simulink model "The_Entire_Control_Algorithm"  (R2024b)
settings: Solver=FixedStepDiscrete  StartTime=0.0  StopTime=10.0  FixedStep=0.001  RelTol=1e-3
undefined symbols (not defined in the file or in its folder): dspblkCoreblockFVToolHelper, gcbh
libraries: arduinolib x21, slpidlib x6, simulink x5, sharedTrackingLibrary x1
(part 1 of 2)
settings Model: Creator=BU  LastModifiedBy=BU
settings OptimizationCC: DefaultParameterBehavior=Inlined  UseDivisionForNetSlopeComputation=on  GainParamInheritBuiltInType=on  UseFloatMulNetSlope=on  InlineInvariantSignals=on  PassReuseOutputArgsAs=Individual arguments  ZeroExternalMemoryAtStartup=off  ZeroInternalMemoryAtStartup=off  NoFixptDivByZeroProtection=on  EfficientFloat2IntCast=on  LifeSpan=1  OptimizeBlockOrder=speed  DifferentSizesBufferReuse=on  EfficientTunableParamExpr=on
settings DebuggingCC: ParameterTunabilityLossMsg=error
settings HardwareCC: ProdBitPerInt=16  ProdBitPerPointer=16  ProdBitPerSizeT=16  ProdBitPerPtrDiffT=16  ProdLargestAtomicFloat=None  ProdWordSize=16  ProdLongLongMode=on  ProdHWDeviceType=Atmel->AVR (8-bit)
settings SFSimCC: MATLABDynamicMemAlloc=off
settings RTWCC: Description=Embedded Coder  SystemTargetFile=ert.tlc  GenCodeOnly=on  TemplateMakefile=ert_default_tmf
settings CodeAppCC: ForceParamTrailComments=on  IgnoreCustomStorageClasses=off  OperatorAnnotations=on  SimulinkDataObjDesc=on  SFDataObjDesc=on  CustomSymbolStrGlobalVar=rt$N$M  CustomSymbolStrType=$N$M  CustomSymbolStrFcn=$N$M$F  CustomSymbolStrMacro=$N$M  InsertBlockDesc=on
settings ERTTargetCC: TargetLangStandard=C99 (ISO)  GenerateSampleERTMain=on  IncludeMdlTerminateFcn=off  CombineSignalStateStructs=on  SupportComplex=off  SupportContinuousTime=on  SupportNonInlinedSFcns=on  RootIOFormat=Structure reference  ERTCustomFileTemplate=example_file_process.tlc  ERTFilePackagingFormat=CompactWithDataFile

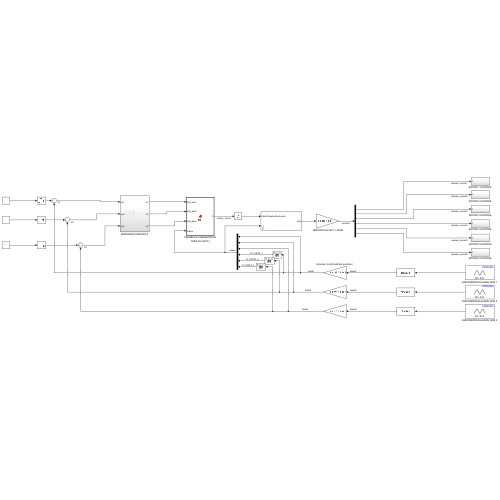
[thumbnail: Simulink's stored preview of the top-level diagram]
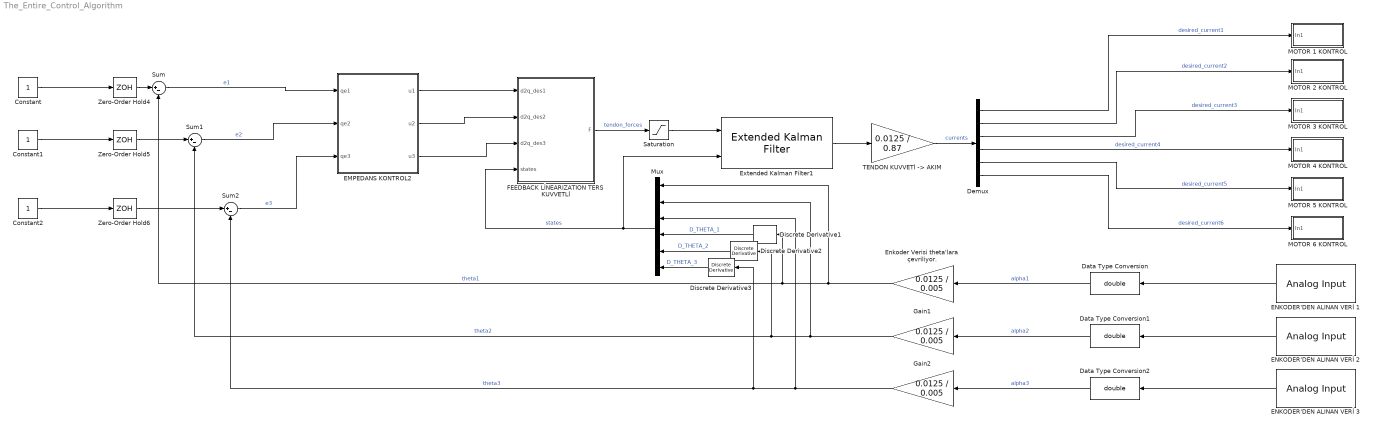
== system The_Entire_Control_Algorithm ==
  Constant : Constant
  Constant1 : Constant
  Constant2 : Constant
  Data Type Conversion : DataTypeConversion  OutDataTypeStr=double  SaturateOnIntegerOverflow=off  RndMeth=Floor
  Data Type Conversion1 : DataTypeConversion  OutDataTypeStr=double  SaturateOnIntegerOverflow=off  RndMeth=Floor
  Data Type Conversion2 : DataTypeConversion  OutDataTypeStr=double  SaturateOnIntegerOverflow=off  RndMeth=Floor
  Demux : Demux  Outputs=6
  Discrete Derivative1 : simulink/Discrete/Discrete Derivative  gainval=1.0  ICPrevScaledInput=0.0  OutMin=[]  OutMax=[]  OutDataType=fixdt(1, 16)  OutScaling=2^-10  DoSatur=off
  Discrete Derivative2 : simulink/Discrete/Discrete Derivative  gainval=1.0  ICPrevScaledInput=0.0  OutMin=[]  OutMax=[]  OutDataType=fixdt(1, 16)  OutScaling=2^-10  DoSatur=off
  Discrete Derivative3 : simulink/Discrete/Discrete Derivative  gainval=1.0  ICPrevScaledInput=0.0  OutMin=[]  OutMax=[]  OutDataType=fixdt(1, 16)  OutScaling=2^-10  DoSatur=off
  EMPEDANS KONTROL2 : Subsystem
  ENKODER'DEN ALINAN VERİ 1 : arduinolib/Analog Input  pinNumber=15  ReadResultsOnly=off  ConversionTriggerSource=Software  ExternalTriggerType=uint32( 0 )  OutputDataType=uint16  EnableConversionCompleteNotify=off  EnableOuputStatus=off  SampleTime=0.001  blockPlatform=arduino
  ENKODER'DEN ALINAN VERİ 2 : arduinolib/Analog Input  pinNumber=14  ReadResultsOnly=off  ConversionTriggerSource=Software  ExternalTriggerType=uint32( 0 )  OutputDataType=uint16  EnableConversionCompleteNotify=off  EnableOuputStatus=off  SampleTime=0.001  blockPlatform=arduino
  ENKODER'DEN ALINAN VERİ 3 : arduinolib/Analog Input  pinNumber=13  ReadResultsOnly=off  ConversionTriggerSource=Software  ExternalTriggerType=uint32( 0 )  OutputDataType=uint16  EnableConversionCompleteNotify=off  EnableOuputStatus=off  SampleTime=0.001  blockPlatform=arduino
  Enkoder Verisi theta'lara çevriliyor. : Gain  Gain=0.0125 / 0.005
  Extended Kalman Filter1 : sharedTrackingLibrary/Extended Kalman Filter  StateTransitionFcn=myStateTransitionFcn  HasStateTransitionJacobianFcn=off  StateTransitionJacobianFcn=0  HasAdditiveProcessNoise=Additive  ProcessNoise=diag([1e-7, 1e-7, 1e-7, 1e-7, 1e-7, 1e-7]);  HasTimeVaryingProcessNoise=off  HasStateTransitionFcnExtraArgument=1  InitialState=[0; 0; 0; 0; 0; 0]  InitialStateCovariance=[1e-6; 1e-6; 1e-6; 1e-6; 1e-6; 1e-6];  MeasurementFcn1=myMeasurementFcn  HasMeasurementJacobianFcn1=off  HasMeasurementEnablePort1=off  HasAdditiveMeasurementNoise1=Additive  MeasurementNoise1=[1e-1; 1e-1; 1e-1; 1e-1; 1e-1; 1e-1];  HasTimeVaryingMeasurementNoise1=off  HasMeasurementFcnExtraArgument1=0  HasMeasurementWrapping1=off  MeasurementFcn2=myMeasurementFcn  HasMeasurementJacobianFcn2=off  HasMeasurementEnablePort2=off  HasAdditiveMeasurementNoise2=Additive  MeasurementNoise2=1  HasTimeVaryingMeasurementNoise2=off  HasMeasurementFcnExtraArgument2=0  HasMeasurementWrapping2=off  MeasurementFcn3=myMeasurementFcn  HasMeasurementJacobianFcn3=off  HasMeasurementEnablePort3=off  HasAdditiveMeasurementNoise3=Additive  MeasurementNoise3=1  HasTimeVaryingMeasurementNoise3=off  HasMeasurementFcnExtraArgument3=0  HasMeasurementWrapping3=off  MeasurementFcn4=myMeasurementFcn  HasMeasurementJacobianFcn4=off  HasMeasurementEnablePort4=off  HasAdditiveMeasurementNoise4=Additive  MeasurementNoise4=1  HasTimeVaryingMeasurementNoise4=off  HasMeasurementFcnExtraArgument4=0  HasMeasurementWrapping4=off  MeasurementFcn5=myMeasurementFcn  HasMeasurementJacobianFcn5=off  HasMeasurementEnablePort5=off  HasAdditiveMeasurementNoise5=Additive  MeasurementNoise5=1  HasTimeVaryingMeasurementNoise5=off  HasMeasurementFcnExtraArgument5=0  HasMeasurementWrapping5=off  EnableMultirate=off  StateTransitionFcnSampleTime=1  MeasurementFcn1SampleTime=1  MeasurementFcn2SampleTime=1  MeasurementFcn3SampleTime=1  MeasurementFcn4SampleTime=1  MeasurementFcn5SampleTime=1  UseCurrentEstimator=on  OutputStateCovariance=off  DataType=double  SampleTime=0.001  NumberOfMeasurements=1
      settings: LibrarySourceBlock=slident/Estimators/Extended Kalman Filter
  FEEDBACK LİNEARIZATION TERS KUVVETLİ : MATLAB Function  TreatAsAtomicUnit=on
  Gain1 : Gain  Gain=0.0125 / 0.005
  Gain2 : Gain  Gain=0.0125 / 0.005
  MOTOR 1 KONTROL : Subsystem
  MOTOR 2 KONTROL : Subsystem
  MOTOR 3 KONTROL : Subsystem
  MOTOR 4 KONTROL : Subsystem
  MOTOR 5 KONTROL : Subsystem
  MOTOR 6 KONTROL : Subsystem
  Mux : Mux  Inputs=6
  Saturation : Saturate  UpperLimit=7  LowerLimit=-7
  Sum : Sum  Inputs=|+-
  Sum1 : Sum  Inputs=|+-
  Sum2 : Sum  Inputs=|+-
  "TENDON KUVVETİ -> AKIM" : Gain  Gain=0.0125 / 0.87
  Zero-Order Hold4 : ZeroOrderHold  SampleTime=0.001
  Zero-Order Hold5 : ZeroOrderHold  SampleTime=0.001
  Zero-Order Hold6 : ZeroOrderHold  SampleTime=0.001
  wires:
  Demux/5 -> MOTOR 5 KONTROL/1(In1)  "desired_current5"
  Demux/4 -> MOTOR 4 KONTROL/1(In1)  "desired_current4"
  Demux/6 -> MOTOR 6 KONTROL/1(In1)  "desired_current6"
  Demux/2 -> MOTOR 2 KONTROL/1(In1)  "desired_current2"
  Demux/3 -> MOTOR 3 KONTROL/1(In1)  "desired_current3"
  ENKODER'DEN ALINAN VERİ 3/1 -> Data Type Conversion2/1
  ENKODER'DEN ALINAN VERİ 1/1 -> Data Type Conversion/1
  ENKODER'DEN ALINAN VERİ 2/1 -> Data Type Conversion1/1
  Demux/1 -> MOTOR 1 KONTROL/1(In1)  "desired_current1"
  Discrete Derivative1/1 -> Mux/4  "D_THETA_1"
  Discrete Derivative2/1 -> Mux/5  "D_THETA_2"
  Discrete Derivative3/1 -> Mux/6  "D_THETA_3"
  Data Type Conversion/1 -> Enkoder Verisi theta'lara çevriliyor./1  "alpha1"
  Data Type Conversion1/1 -> Gain1/1  "alpha2"
  Data Type Conversion2/1 -> Gain2/1  "alpha3"
  "TENDON KUVVETİ -> AKIM"/1 -> Demux/1  "currents"
  Enkoder Verisi theta'lara çevriliyor./1 -> Sum/2, Discrete Derivative1/1, Mux/1  "theta1"
  Gain1/1 -> Sum1/2, Discrete Derivative2/1, Mux/2  "theta2"
  Gain2/1 -> Sum2/2, Discrete Derivative3/1, Mux/3  "theta3"
  Zero-Order Hold4/1 -> Sum/1
  EMPEDANS KONTROL2/2(u2) -> FEEDBACK LİNEARIZATION TERS KUVVETLİ/2(d2q_des2)
  Sum/1 -> EMPEDANS KONTROL2/1(qe1)  "e1"
  Sum1/1 -> EMPEDANS KONTROL2/2(qe2)  "e2"
  Sum2/1 -> EMPEDANS KONTROL2/3(qe3)  "e3"
  Zero-Order Hold6/1 -> Sum2/1
  Constant1/1 -> Zero-Order Hold5/1
  FEEDBACK LİNEARIZATION TERS KUVVETLİ/1(F) -> Saturation/1  "tendon_forces"
  Zero-Order Hold5/1 -> Sum1/1
  EMPEDANS KONTROL2/1(u1) -> FEEDBACK LİNEARIZATION TERS KUVVETLİ/1(d2q_des1)
  Constant2/1 -> Zero-Order Hold6/1
  EMPEDANS KONTROL2/3(u3) -> FEEDBACK LİNEARIZATION TERS KUVVETLİ/3(d2q_des3)
  Constant/1 -> Zero-Order Hold4/1
  Mux/1 -> Extended Kalman Filter1/2, FEEDBACK LİNEARIZATION TERS KUVVETLİ/4(states)  "states"
  Saturation/1 -> Extended Kalman Filter1/1
  Extended Kalman Filter1/1 -> "TENDON KUVVETİ -> AKIM"/1

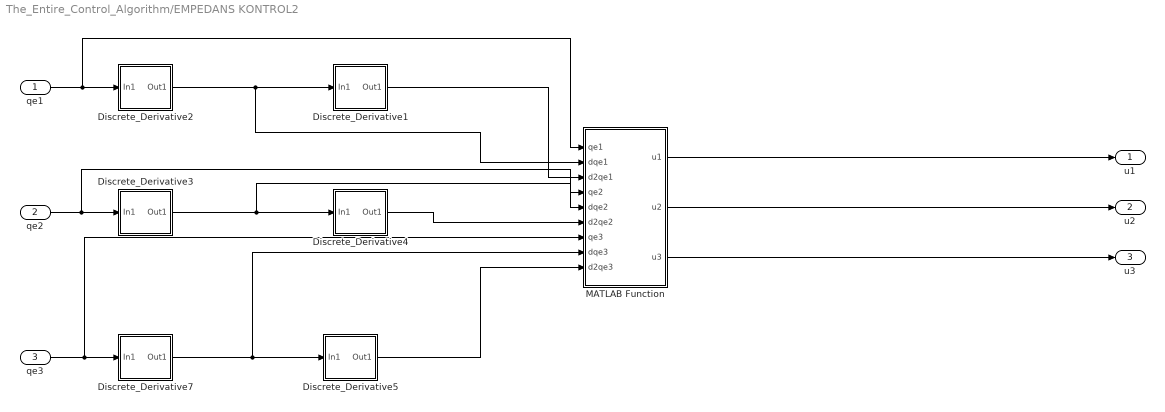
== system The_Entire_Control_Algorithm/EMPEDANS KONTROL2 ==
  qe1 : Inport
  qe2 : Inport  Port=2
  qe3 : Inport  Port=3
  Discrete_Derivative1 : Subsystem
  Discrete_Derivative2 : Subsystem
  Discrete_Derivative3 : Subsystem
  Discrete_Derivative4 : Subsystem
  Discrete_Derivative5 : Subsystem
  Discrete_Derivative7 : Subsystem
  MATLAB Function : MATLAB Function  TreatAsAtomicUnit=on
  u1 : Outport
  u2 : Outport  Port=2
  u3 : Outport  Port=3
  wires:
  qe1/1 -> Discrete_Derivative2/1(In1), MATLAB Function/1(qe1)
  qe2/1 -> Discrete_Derivative3/1(In1), MATLAB Function/4(qe2)
  qe3/1 -> Discrete_Derivative7/1(In1), MATLAB Function/7(qe3)
  Discrete_Derivative2/1(Out1) -> Discrete_Derivative1/1(In1), MATLAB Function/2(dqe1)
  Discrete_Derivative3/1(Out1) -> Discrete_Derivative4/1(In1), MATLAB Function/5(dqe2)
  Discrete_Derivative7/1(Out1) -> Discrete_Derivative5/1(In1), MATLAB Function/8(dqe3)
  Discrete_Derivative1/1(Out1) -> MATLAB Function/3(d2qe1)
  Discrete_Derivative4/1(Out1) -> MATLAB Function/6(d2qe2)
  Discrete_Derivative5/1(Out1) -> MATLAB Function/9(d2qe3)
  MATLAB Function/1(u1) -> u1/1
  MATLAB Function/2(u2) -> u2/1
  MATLAB Function/3(u3) -> u3/1

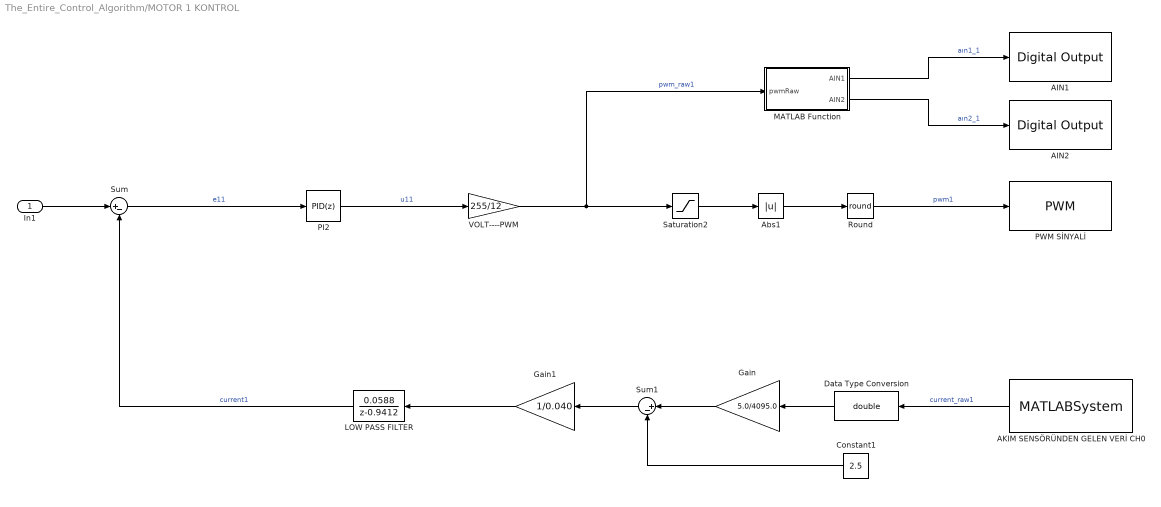
== system The_Entire_Control_Algorithm/MOTOR 1 KONTROL ==
  In1 : Inport
  AIN1 : arduinolib/Digital Output  pinNumber=24  Direction=output  blockPlatform=arduino
  AIN2 : arduinolib/Digital Output  pinNumber=25  Direction=output  blockPlatform=arduino
  AKIM SENSÖRÜNDEN GELEN VERİ CH0 : MATLABSystem  System=MCP3208Reader  Channel=0  SimulateUsing=Code generation
      mask Type: MCP3208Reader
      mask Display:
      | disp('MCP3208Reader');
      | port_label('output',1,'value');
  Abs1 : Abs  RndMeth=Round  SaturateOnIntegerOverflow=off
  Constant1 : Constant  Value=2.5
  Data Type Conversion : DataTypeConversion  OutDataTypeStr=double  SaturateOnIntegerOverflow=off  RndMeth=Floor
  Gain : Gain  Gain=5.0/4095.0
  Gain1 : Gain  Gain=1/0.040
  LOW PASS FILTER : DiscreteTransferFcn  LoadFcn=dspblkCoreblockFVToolHelper(gcbh,'load');  Numerator=[0.0588]  Denominator=[1 -0.9412]
      settings: CopyFcn=dspblkCoreblockFVToolHelper(gcbh,'copy');  DeleteFcn=dspblkCoreblockFVToolHelper(gcbh,'close');  ModelCloseFcn=dspblkCoreblockFVToolHelper(gcbh,'close');  PreSaveFcn=dspblkCoreblockFVToolHelper(gcbh,'presave');  PostSaveFcn=dspblkCoreblockFVToolHelper(gcbh,'postsave');  CloseFcn=dspblkCoreblockFVToolHelper(gcbh,'close');
  MATLAB Function : MATLAB Function  TreatAsAtomicUnit=on
  PI2 : slpidlib/PID Controller  Controller=PID  Form=Parallel  TimeDomain=Discrete-time  UseExternalTs=off  SampleTime=0.001  IntegratorMethod=Forward Euler  FilterMethod=Forward Euler  ControllerParametersSource=internal  P=21  I=900  UseKiTs=off  D=0  UseExternalDerivativeSource=off  N=100  UseFilter=off  TunerSelectOption=Transfer Function Based (PID Tuner App)  InitialConditionSource=internal  InitialConditionForIntegrator=0  InitialConditionForFilter=0  DifferentiatorICPrevScaledInput=0  ExternalReset=none  TrackingMode=off  Kt=1  LimitOutput=off  SatLimitsSource=internal  UpperSaturationLimit=inf  LowerSaturationLimit=-inf  LinearizeAsGain=on  AntiWindupMode=none  Kb=1  LimitIntegrator=off  UpperIntegratorSaturationLimit=inf  LowerIntegratorSaturationLimit=-inf  POutMin=[]  POutMax=[]  IOutMin=[]  IOutMax=[]  DOutMin=[]  DOutMax=[]  NOutMin=[]  NOutMax=[]  SumOutMin=[]  SumOutMax=[]  SaturationOutMin=[]  SaturationOutMax=[]  PParamMin=[]  PParamMax=[]  IParamMin=[]  IParamMax=[]  DParamMin=[]  DParamMax=[]  NParamMin=[]  NParamMax=[]  KbParamMin=[]  KbParamMax=[]  KtParamMin=[]  KtParamMax=[]  KbOutMin=[]  KbOutMax=[]  KtOutMin=[]  KtOutMax=[]  IntegratorOutMin=[]  IntegratorOutMax=[]  FilterOutMin=[]  FilterOutMax=[]  SumI1OutMin=[]  SumI1OutMax=[]  SumI2OutMin=[]  SumI2OutMax=[]  SumI3OutMin=[]  SumI3OutMax=[]  SumI4OutMin=[]  SumI4OutMax=[]  SumDOutMin=[]  SumDOutMax=[]  DifferentiatorOutMin=[]  DifferentiatorOutMax=[]  FilterDiffOutCoefMin=[]  FilterDiffOutCoefMax=[]  ReciprocalOutMin=[]  ReciprocalOutMax=[]  SumDenOutMin=[]  SumDenOutMax=[]  SumNumOutMin=[]  SumNumOutMax=[]  DivideOutMin=[]  DivideOutMax=[]  UdiffTsProdOutMin=[]  UdiffTsProdOutMax=[]  NTsProdOutMin=[]  NTsProdOutMax=[]  UintegralTsProdOutMin=[]  UintegralTsProdOutMax=[]  UngainTsProdOutMin=[]  UngainTsProdOutMax=[]  ClampingZeroOutDataTypeStr=Inherit: Inherit via back propagation  ClampingZeroOutMin=[]  ClampingZeroOutMax=[]  FilterDenConstantOutDataTypeStr=Inherit: Inherit via back propagation  FilterDenConstantOutMin=[]  FilterDenConstantOutMax=[]  PCopyOutDataTypeStr=Inherit: Inherit via back propagation  PCopyOutMin=[]  PCopyOutMax=[]  NCopyOutDataTypeStr=Inherit: Inherit via back propagation  NCopyOutMin=[]  NCopyOutMax=[]  IntegratorContinuousStateAttributes=''  IntegratorStateMustResolveToSignalObject=off  IntegratorRTWStateStorageClass=Auto  FilterContinuousStateAttributes=''  FilterStateMustResolveToSignalObject=off  FilterRTWStateStorageClass=Auto  ParallelPVariant=InternalParameters  IdealPVariant=Disabled  IVariant=InternalParameters  DVariant=InternalParameters  IntegratorVariant=Discrete  SatVariant=Disabled  AWVariant=Passthrough  PCopyVariant=Disabled  TRVariant=Disabled  FdbkBlocksVariant=Forward  IdealPFdbkVariant=Disabled  SatFdbkVariant=Disabled  DerivativeFilterVariant=Differentiator  NVariant=Passthrough  NCopyVariant=Disabled_SignalSpec  FilterICVariant=InternalICsDifferentiator  IntegratorICVariant=InternalICs  ExternalResetVariant=Disabled  TRSumVariant=Passthrough  SumFdbkVariant=Disabled  SumVariant=Sum_PID  TsampFilterVariant=InternalTs  TsampNgainVariant=Passthrough  TsampIntegralVariant=Disabled_SignalSpec  ExternalSaturationOutDataTypeStr=Inherit: Same as second input  DerivativeSourceVariant=ErrorSignal  PreIntVariant=InternalPreInt
  PWM SİNYALİ : arduinolib/PWM  pinNumber=2  frequencyType=Default  desiredFrequency=490  achievableFrequency=490.2
  Round : Rounding  Operator=round
  Saturation2 : Saturate  UpperLimit=255  LowerLimit=-255
  Sum : Sum  Inputs=|+-
  Sum1 : Sum  Inputs=|+-
  VOLT----PWM : Gain  Gain=255/12
  wires:
  Gain1/1 -> LOW PASS FILTER/1
  VOLT----PWM/1 -> MATLAB Function/1(pwmRaw), Saturation2/1  "pwm_raw1"
  MATLAB Function/2(AIN2) -> AIN2/1  "aın2_1"
  Saturation2/1 -> Abs1/1
  Sum1/1 -> Gain1/1
  PI2/1 -> VOLT----PWM/1  "u11"
  In1/1 -> Sum/1
  LOW PASS FILTER/1 -> Sum/2  "current1"
  Round/1 -> PWM SİNYALİ/1  "pwm1"
  Constant1/1 -> Sum1/2
  AKIM SENSÖRÜNDEN GELEN VERİ CH0/1 -> Data Type Conversion/1  "current_raw1"
  Gain/1 -> Sum1/1
  Abs1/1 -> Round/1
  Sum/1 -> PI2/1  "e11"
  MATLAB Function/1(AIN1) -> AIN1/1  "aın1_1"
  Data Type Conversion/1 -> Gain/1

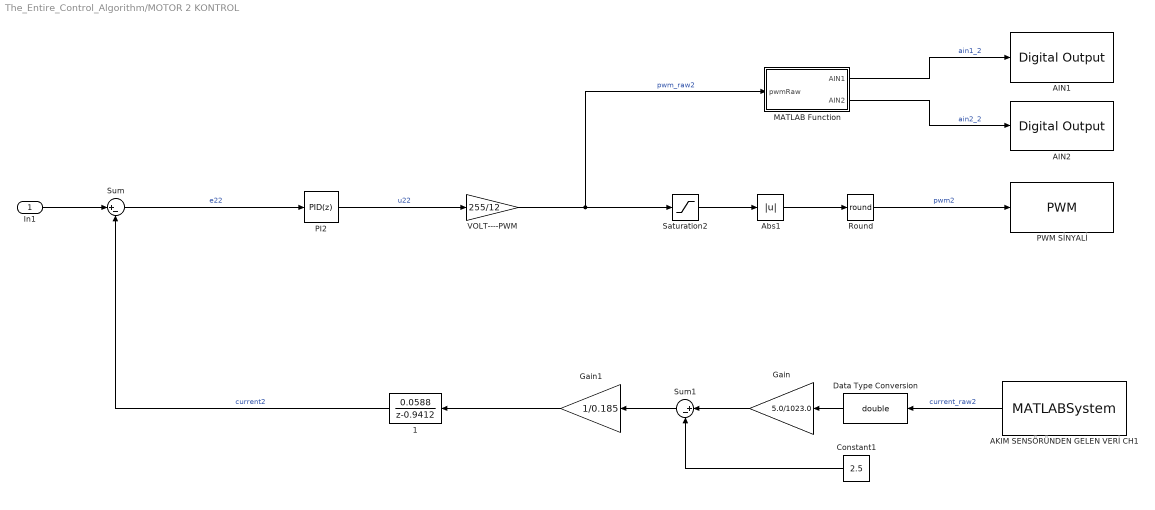
== system The_Entire_Control_Algorithm/MOTOR 2 KONTROL ==
  In1 : Inport
  1 : DiscreteTransferFcn  LoadFcn=dspblkCoreblockFVToolHelper(gcbh,'load');  Numerator=[0.0588]  Denominator=[1 -0.9412]
      settings: CopyFcn=dspblkCoreblockFVToolHelper(gcbh,'copy');  DeleteFcn=dspblkCoreblockFVToolHelper(gcbh,'close');  ModelCloseFcn=dspblkCoreblockFVToolHelper(gcbh,'close');  PreSaveFcn=dspblkCoreblockFVToolHelper(gcbh,'presave');  PostSaveFcn=dspblkCoreblockFVToolHelper(gcbh,'postsave');  CloseFcn=dspblkCoreblockFVToolHelper(gcbh,'close');
  AIN1 : arduinolib/Digital Output  pinNumber=26  Direction=output  blockPlatform=arduino
  AIN2 : arduinolib/Digital Output  pinNumber=27  Direction=output  blockPlatform=arduino
  AKIM SENSÖRÜNDEN GELEN VERİ CH1 : MATLABSystem  System=MCP3208Reader  Channel=0  SimulateUsing=Code generation
      mask Type: MCP3208Reader
      mask Display:
      | disp('MCP3208Reader');
      | port_label('output',1,'value');
  Abs1 : Abs  RndMeth=Round  SaturateOnIntegerOverflow=off
  Constant1 : Constant  Value=2.5
  Data Type Conversion : DataTypeConversion  OutDataTypeStr=double  SaturateOnIntegerOverflow=off  RndMeth=Floor
  Gain : Gain  Gain=5.0/1023.0
  Gain1 : Gain  Gain=1/0.185
  MATLAB Function : MATLAB Function  TreatAsAtomicUnit=on
  PI2 : slpidlib/PID Controller  Controller=PID  Form=Parallel  TimeDomain=Discrete-time  UseExternalTs=off  SampleTime=0.001  IntegratorMethod=Forward Euler  FilterMethod=Forward Euler  ControllerParametersSource=internal  P=21  I=900  UseKiTs=off  D=0.15  UseExternalDerivativeSource=off  N=100  UseFilter=off  TunerSelectOption=Transfer Function Based (PID Tuner App)  InitialConditionSource=internal  InitialConditionForIntegrator=0  InitialConditionForFilter=0  DifferentiatorICPrevScaledInput=0  ExternalReset=none  TrackingMode=off  Kt=1  LimitOutput=off  SatLimitsSource=internal  UpperSaturationLimit=inf  LowerSaturationLimit=-inf  LinearizeAsGain=on  AntiWindupMode=none  Kb=1  LimitIntegrator=off  UpperIntegratorSaturationLimit=inf  LowerIntegratorSaturationLimit=-inf  POutMin=[]  POutMax=[]  IOutMin=[]  IOutMax=[]  DOutMin=[]  DOutMax=[]  NOutMin=[]  NOutMax=[]  SumOutMin=[]  SumOutMax=[]  SaturationOutMin=[]  SaturationOutMax=[]  PParamMin=[]  PParamMax=[]  IParamMin=[]  IParamMax=[]  DParamMin=[]  DParamMax=[]  NParamMin=[]  NParamMax=[]  KbParamMin=[]  KbParamMax=[]  KtParamMin=[]  KtParamMax=[]  KbOutMin=[]  KbOutMax=[]  KtOutMin=[]  KtOutMax=[]  IntegratorOutMin=[]  IntegratorOutMax=[]  FilterOutMin=[]  FilterOutMax=[]  SumI1OutMin=[]  SumI1OutMax=[]  SumI2OutMin=[]  SumI2OutMax=[]  SumI3OutMin=[]  SumI3OutMax=[]  SumI4OutMin=[]  SumI4OutMax=[]  SumDOutMin=[]  SumDOutMax=[]  DifferentiatorOutMin=[]  DifferentiatorOutMax=[]  FilterDiffOutCoefMin=[]  FilterDiffOutCoefMax=[]  ReciprocalOutMin=[]  ReciprocalOutMax=[]  SumDenOutMin=[]  SumDenOutMax=[]  SumNumOutMin=[]  SumNumOutMax=[]  DivideOutMin=[]  DivideOutMax=[]  UdiffTsProdOutMin=[]  UdiffTsProdOutMax=[]  NTsProdOutMin=[]  NTsProdOutMax=[]  UintegralTsProdOutMin=[]  UintegralTsProdOutMax=[]  UngainTsProdOutMin=[]  UngainTsProdOutMax=[]  ClampingZeroOutDataTypeStr=Inherit: Inherit via back propagation  ClampingZeroOutMin=[]  ClampingZeroOutMax=[]  FilterDenConstantOutDataTypeStr=Inherit: Inherit via back propagation  FilterDenConstantOutMin=[]  FilterDenConstantOutMax=[]  PCopyOutDataTypeStr=Inherit: Inherit via back propagation  PCopyOutMin=[]  PCopyOutMax=[]  NCopyOutDataTypeStr=Inherit: Inherit via back propagation  NCopyOutMin=[]  NCopyOutMax=[]  IntegratorContinuousStateAttributes=''  IntegratorStateMustResolveToSignalObject=off  IntegratorRTWStateStorageClass=Auto  FilterContinuousStateAttributes=''  FilterStateMustResolveToSignalObject=off  FilterRTWStateStorageClass=Auto  ParallelPVariant=InternalParameters  IdealPVariant=Disabled  IVariant=InternalParameters  DVariant=InternalParameters  IntegratorVariant=Discrete  SatVariant=Disabled  AWVariant=Passthrough  PCopyVariant=Disabled  TRVariant=Disabled  FdbkBlocksVariant=Forward  IdealPFdbkVariant=Disabled  SatFdbkVariant=Disabled  DerivativeFilterVariant=Differentiator  NVariant=Passthrough  NCopyVariant=Disabled_SignalSpec  FilterICVariant=InternalICsDifferentiator  IntegratorICVariant=InternalICs  ExternalResetVariant=Disabled  TRSumVariant=Passthrough  SumFdbkVariant=Disabled  SumVariant=Sum_PID  TsampFilterVariant=InternalTs  TsampNgainVariant=Passthrough  TsampIntegralVariant=Disabled_SignalSpec  ExternalSaturationOutDataTypeStr=Inherit: Same as second input  DerivativeSourceVariant=ErrorSignal  PreIntVariant=InternalPreInt
  PWM SİNYALİ : arduinolib/PWM  pinNumber=3  frequencyType=Specify  desiredFrequency=490  achievableFrequency=490.2
  Round : Rounding  Operator=round
  Saturation2 : Saturate  UpperLimit=255  LowerLimit=-255
  Sum : Sum  Inputs=|+-
  Sum1 : Sum  Inputs=|+-
  VOLT----PWM : Gain  Gain=255/12
  wires:
  In1/1 -> Sum/1
  MATLAB Function/1(AIN1) -> AIN1/1  "ain1_2"
  Sum/1 -> PI2/1  "e22"
  Constant1/1 -> Sum1/2
  Round/1 -> PWM SİNYALİ/1  "pwm2"
  Gain/1 -> Sum1/1
  Abs1/1 -> Round/1
  1/1 -> Sum/2  "current2"
  VOLT----PWM/1 -> MATLAB Function/1(pwmRaw), Saturation2/1  "pwm_raw2"
  MATLAB Function/2(AIN2) -> AIN2/1  "ain2_2"
  Saturation2/1 -> Abs1/1
  Gain1/1 -> 1/1
  Sum1/1 -> Gain1/1
  PI2/1 -> VOLT----PWM/1  "u22"
  Data Type Conversion/1 -> Gain/1
  AKIM SENSÖRÜNDEN GELEN VERİ CH1/1 -> Data Type Conversion/1  "current_raw2"

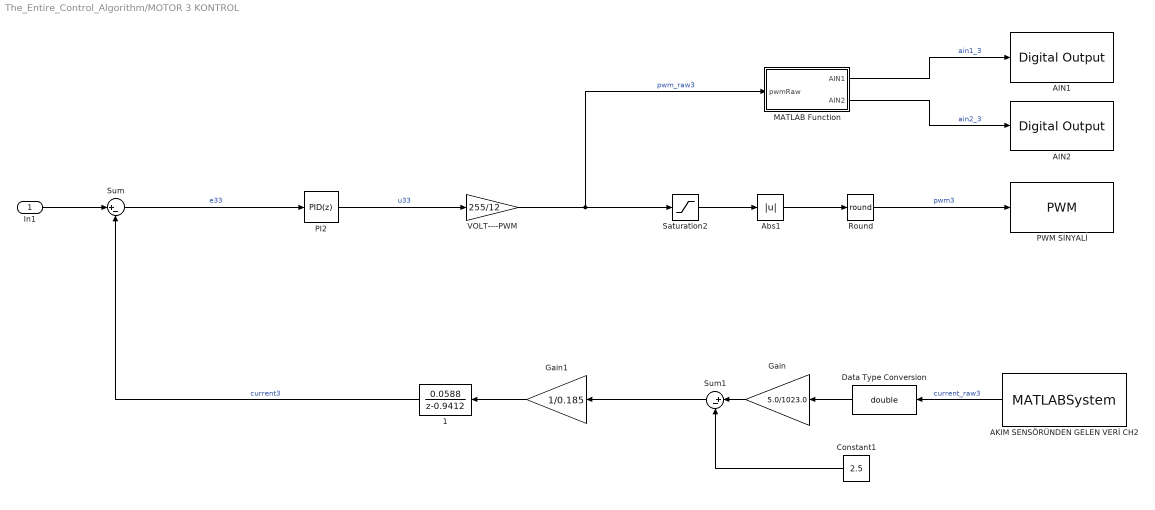
== system The_Entire_Control_Algorithm/MOTOR 3 KONTROL ==
  In1 : Inport
  1 : DiscreteTransferFcn  LoadFcn=dspblkCoreblockFVToolHelper(gcbh,'load');  Numerator=[0.0588]  Denominator=[1 -0.9412]
      settings: CopyFcn=dspblkCoreblockFVToolHelper(gcbh,'copy');  DeleteFcn=dspblkCoreblockFVToolHelper(gcbh,'close');  ModelCloseFcn=dspblkCoreblockFVToolHelper(gcbh,'close');  PreSaveFcn=dspblkCoreblockFVToolHelper(gcbh,'presave');  PostSaveFcn=dspblkCoreblockFVToolHelper(gcbh,'postsave');  CloseFcn=dspblkCoreblockFVToolHelper(gcbh,'close');
  AIN1 : arduinolib/Digital Output  pinNumber=28  Direction=output  blockPlatform=arduino
  AIN2 : arduinolib/Digital Output  pinNumber=29  Direction=output  blockPlatform=arduino
  AKIM SENSÖRÜNDEN GELEN VERİ CH2 : MATLABSystem  System=MCP3208Reader  Channel=0  SimulateUsing=Code generation
      mask Type: MCP3208Reader
      mask Display:
      | disp('MCP3208Reader');
      | port_label('output',1,'value');
  Abs1 : Abs  RndMeth=Round  SaturateOnIntegerOverflow=off
  Constant1 : Constant  Value=2.5
  Data Type Conversion : DataTypeConversion  OutDataTypeStr=double  SaturateOnIntegerOverflow=off  RndMeth=Floor
  Gain : Gain  Gain=5.0/1023.0
  Gain1 : Gain  Gain=1/0.185
  MATLAB Function : MATLAB Function  TreatAsAtomicUnit=on
  PI2 : slpidlib/PID Controller  Controller=PID  Form=Parallel  TimeDomain=Discrete-time  UseExternalTs=off  SampleTime=0.001  IntegratorMethod=Forward Euler  FilterMethod=Forward Euler  ControllerParametersSource=internal  P=21  I=900  UseKiTs=off  D=0.15  UseExternalDerivativeSource=off  N=100  UseFilter=off  TunerSelectOption=Transfer Function Based (PID Tuner App)  InitialConditionSource=internal  InitialConditionForIntegrator=0  InitialConditionForFilter=0  DifferentiatorICPrevScaledInput=0  ExternalReset=none  TrackingMode=off  Kt=1  LimitOutput=off  SatLimitsSource=internal  UpperSaturationLimit=inf  LowerSaturationLimit=-inf  LinearizeAsGain=on  AntiWindupMode=none  Kb=1  LimitIntegrator=off  UpperIntegratorSaturationLimit=inf  LowerIntegratorSaturationLimit=-inf  POutMin=[]  POutMax=[]  IOutMin=[]  IOutMax=[]  DOutMin=[]  DOutMax=[]  NOutMin=[]  NOutMax=[]  SumOutMin=[]  SumOutMax=[]  SaturationOutMin=[]  SaturationOutMax=[]  PParamMin=[]  PParamMax=[]  IParamMin=[]  IParamMax=[]  DParamMin=[]  DParamMax=[]  NParamMin=[]  NParamMax=[]  KbParamMin=[]  KbParamMax=[]  KtParamMin=[]  KtParamMax=[]  KbOutMin=[]  KbOutMax=[]  KtOutMin=[]  KtOutMax=[]  IntegratorOutMin=[]  IntegratorOutMax=[]  FilterOutMin=[]  FilterOutMax=[]  SumI1OutMin=[]  SumI1OutMax=[]  SumI2OutMin=[]  SumI2OutMax=[]  SumI3OutMin=[]  SumI3OutMax=[]  SumI4OutMin=[]  SumI4OutMax=[]  SumDOutMin=[]  SumDOutMax=[]  DifferentiatorOutMin=[]  DifferentiatorOutMax=[]  FilterDiffOutCoefMin=[]  FilterDiffOutCoefMax=[]  ReciprocalOutMin=[]  ReciprocalOutMax=[]  SumDenOutMin=[]  SumDenOutMax=[]  SumNumOutMin=[]  SumNumOutMax=[]  DivideOutMin=[]  DivideOutMax=[]  UdiffTsProdOutMin=[]  UdiffTsProdOutMax=[]  NTsProdOutMin=[]  NTsProdOutMax=[]  UintegralTsProdOutMin=[]  UintegralTsProdOutMax=[]  UngainTsProdOutMin=[]  UngainTsProdOutMax=[]  ClampingZeroOutDataTypeStr=Inherit: Inherit via back propagation  ClampingZeroOutMin=[]  ClampingZeroOutMax=[]  FilterDenConstantOutDataTypeStr=Inherit: Inherit via back propagation  FilterDenConstantOutMin=[]  FilterDenConstantOutMax=[]  PCopyOutDataTypeStr=Inherit: Inherit via back propagation  PCopyOutMin=[]  PCopyOutMax=[]  NCopyOutDataTypeStr=Inherit: Inherit via back propagation  NCopyOutMin=[]  NCopyOutMax=[]  IntegratorContinuousStateAttributes=''  IntegratorStateMustResolveToSignalObject=off  IntegratorRTWStateStorageClass=Auto  FilterContinuousStateAttributes=''  FilterStateMustResolveToSignalObject=off  FilterRTWStateStorageClass=Auto  ParallelPVariant=InternalParameters  IdealPVariant=Disabled  IVariant=InternalParameters  DVariant=InternalParameters  IntegratorVariant=Discrete  SatVariant=Disabled  AWVariant=Passthrough  PCopyVariant=Disabled  TRVariant=Disabled  FdbkBlocksVariant=Forward  IdealPFdbkVariant=Disabled  SatFdbkVariant=Disabled  DerivativeFilterVariant=Differentiator  NVariant=Passthrough  NCopyVariant=Disabled_SignalSpec  FilterICVariant=InternalICsDifferentiator  IntegratorICVariant=InternalICs  ExternalResetVariant=Disabled  TRSumVariant=Passthrough  SumFdbkVariant=Disabled  SumVariant=Sum_PID  TsampFilterVariant=InternalTs  TsampNgainVariant=Passthrough  TsampIntegralVariant=Disabled_SignalSpec  ExternalSaturationOutDataTypeStr=Inherit: Same as second input  DerivativeSourceVariant=ErrorSignal  PreIntVariant=InternalPreInt
  PWM SİNYALİ : arduinolib/PWM  pinNumber=4  frequencyType=Default  desiredFrequency=490  achievableFrequency=490.2
  Round : Rounding  Operator=round
  Saturation2 : Saturate  UpperLimit=255  LowerLimit=-255
  Sum : Sum  Inputs=|+-
  Sum1 : Sum  Inputs=|+-
  VOLT----PWM : Gain  Gain=255/12
  wires:
  In1/1 -> Sum/1
  Gain1/1 -> 1/1
  Saturation2/1 -> Abs1/1
  PI2/1 -> VOLT----PWM/1  "u33"
  MATLAB Function/2(AIN2) -> AIN2/1  "ain2_3"
  Sum1/1 -> Gain1/1
  Gain/1 -> Sum1/1
  VOLT----PWM/1 -> MATLAB Function/1(pwmRaw), Saturation2/1  "pwm_raw3"
  Abs1/1 -> Round/1
  1/1 -> Sum/2  "current3"
  Sum/1 -> PI2/1  "e33"
  Round/1 -> PWM SİNYALİ/1  "pwm3"
  Constant1/1 -> Sum1/2
  MATLAB Function/1(AIN1) -> AIN1/1  "ain1_3"
  Data Type Conversion/1 -> Gain/1
  AKIM SENSÖRÜNDEN GELEN VERİ CH2/1 -> Data Type Conversion/1  "current_raw3"

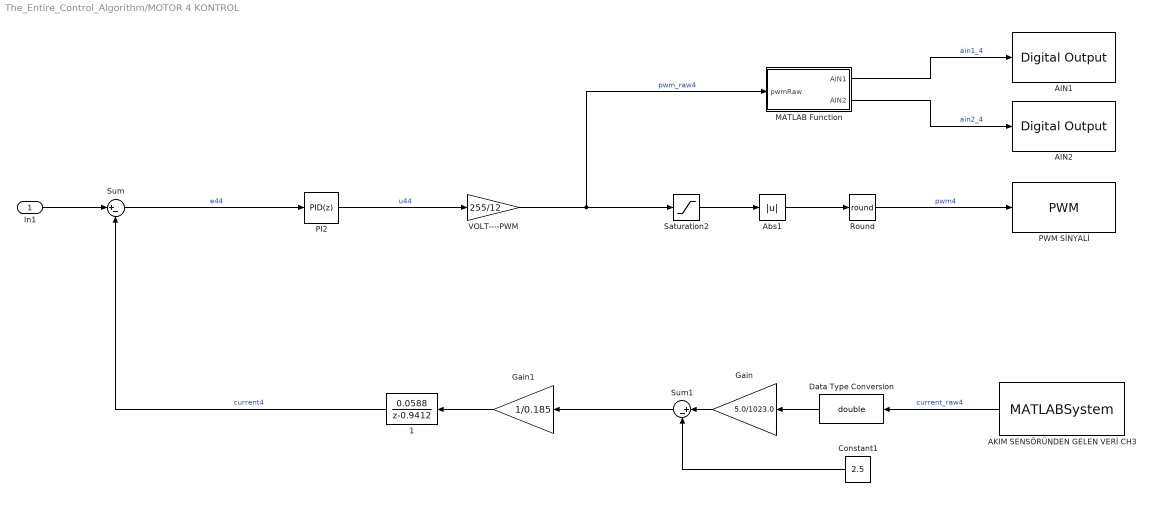
== system The_Entire_Control_Algorithm/MOTOR 4 KONTROL ==
  In1 : Inport
  1 : DiscreteTransferFcn  LoadFcn=dspblkCoreblockFVToolHelper(gcbh,'load');  Numerator=[0.0588]  Denominator=[1 -0.9412]
      settings: CopyFcn=dspblkCoreblockFVToolHelper(gcbh,'copy');  DeleteFcn=dspblkCoreblockFVToolHelper(gcbh,'close');  ModelCloseFcn=dspblkCoreblockFVToolHelper(gcbh,'close');  PreSaveFcn=dspblkCoreblockFVToolHelper(gcbh,'presave');  PostSaveFcn=dspblkCoreblockFVToolHelper(gcbh,'postsave');  CloseFcn=dspblkCoreblockFVToolHelper(gcbh,'close');
  AIN1 : arduinolib/Digital Output  pinNumber=30  Direction=output  blockPlatform=arduino
  AIN2 : arduinolib/Digital Output  pinNumber=31  Direction=output  blockPlatform=arduino
  AKIM SENSÖRÜNDEN GELEN VERİ CH3 : MATLABSystem  System=MCP3208Reader  Channel=0  SimulateUsing=Code generation
      mask Type: MCP3208Reader
      mask Display:
      | disp('MCP3208Reader');
      | port_label('output',1,'value');
  Abs1 : Abs  RndMeth=Round  SaturateOnIntegerOverflow=off
  Constant1 : Constant  Value=2.5
  Data Type Conversion : DataTypeConversion  OutDataTypeStr=double  SaturateOnIntegerOverflow=off  RndMeth=Floor
  Gain : Gain  Gain=5.0/1023.0
  Gain1 : Gain  Gain=1/0.185
  MATLAB Function : MATLAB Function  TreatAsAtomicUnit=on
  PI2 : slpidlib/PID Controller  Controller=PID  Form=Parallel  TimeDomain=Discrete-time  UseExternalTs=off  SampleTime=0.001  IntegratorMethod=Forward Euler  FilterMethod=Forward Euler  ControllerParametersSource=internal  P=21  I=900  UseKiTs=off  D=0.15  UseExternalDerivativeSource=off  N=100  UseFilter=off  TunerSelectOption=Transfer Function Based (PID Tuner App)  InitialConditionSource=internal  InitialConditionForIntegrator=0  InitialConditionForFilter=0  DifferentiatorICPrevScaledInput=0  ExternalReset=none  TrackingMode=off  Kt=1  LimitOutput=off  SatLimitsSource=internal  UpperSaturationLimit=inf  LowerSaturationLimit=-inf  LinearizeAsGain=on  AntiWindupMode=none  Kb=1  LimitIntegrator=off  UpperIntegratorSaturationLimit=inf  LowerIntegratorSaturationLimit=-inf  POutMin=[]  POutMax=[]  IOutMin=[]  IOutMax=[]  DOutMin=[]  DOutMax=[]  NOutMin=[]  NOutMax=[]  SumOutMin=[]  SumOutMax=[]  SaturationOutMin=[]  SaturationOutMax=[]  PParamMin=[]  PParamMax=[]  IParamMin=[]  IParamMax=[]  DParamMin=[]  DParamMax=[]  NParamMin=[]  NParamMax=[]  KbParamMin=[]  KbParamMax=[]  KtParamMin=[]  KtParamMax=[]  KbOutMin=[]  KbOutMax=[]  KtOutMin=[]  KtOutMax=[]  IntegratorOutMin=[]  IntegratorOutMax=[]  FilterOutMin=[]  FilterOutMax=[]  SumI1OutMin=[]  SumI1OutMax=[]  SumI2OutMin=[]  SumI2OutMax=[]  SumI3OutMin=[]  SumI3OutMax=[]  SumI4OutMin=[]  SumI4OutMax=[]  SumDOutMin=[]  SumDOutMax=[]  DifferentiatorOutMin=[]  DifferentiatorOutMax=[]  FilterDiffOutCoefMin=[]  FilterDiffOutCoefMax=[]  ReciprocalOutMin=[]  ReciprocalOutMax=[]  SumDenOutMin=[]  SumDenOutMax=[]  SumNumOutMin=[]  SumNumOutMax=[]  DivideOutMin=[]  DivideOutMax=[]  UdiffTsProdOutMin=[]  UdiffTsProdOutMax=[]  NTsProdOutMin=[]  NTsProdOutMax=[]  UintegralTsProdOutMin=[]  UintegralTsProdOutMax=[]  UngainTsProdOutMin=[]  UngainTsProdOutMax=[]  ClampingZeroOutDataTypeStr=Inherit: Inherit via back propagation  ClampingZeroOutMin=[]  ClampingZeroOutMax=[]  FilterDenConstantOutDataTypeStr=Inherit: Inherit via back propagation  FilterDenConstantOutMin=[]  FilterDenConstantOutMax=[]  PCopyOutDataTypeStr=Inherit: Inherit via back propagation  PCopyOutMin=[]  PCopyOutMax=[]  NCopyOutDataTypeStr=Inherit: Inherit via back propagation  NCopyOutMin=[]  NCopyOutMax=[]  IntegratorContinuousStateAttributes=''  IntegratorStateMustResolveToSignalObject=off  IntegratorRTWStateStorageClass=Auto  FilterContinuousStateAttributes=''  FilterStateMustResolveToSignalObject=off  FilterRTWStateStorageClass=Auto  ParallelPVariant=InternalParameters  IdealPVariant=Disabled  IVariant=InternalParameters  DVariant=InternalParameters  IntegratorVariant=Discrete  SatVariant=Disabled  AWVariant=Passthrough  PCopyVariant=Disabled  TRVariant=Disabled  FdbkBlocksVariant=Forward  IdealPFdbkVariant=Disabled  SatFdbkVariant=Disabled  DerivativeFilterVariant=Differentiator  NVariant=Passthrough  NCopyVariant=Disabled_SignalSpec  FilterICVariant=InternalICsDifferentiator  IntegratorICVariant=InternalICs  ExternalResetVariant=Disabled  TRSumVariant=Passthrough  SumFdbkVariant=Disabled  SumVariant=Sum_PID  TsampFilterVariant=InternalTs  TsampNgainVariant=Passthrough  TsampIntegralVariant=Disabled_SignalSpec  ExternalSaturationOutDataTypeStr=Inherit: Same as second input  DerivativeSourceVariant=ErrorSignal  PreIntVariant=InternalPreInt
  PWM SİNYALİ : arduinolib/PWM  pinNumber=5  frequencyType=Default  desiredFrequency=490  achievableFrequency=490.2
  Round : Rounding  Operator=round
  Saturation2 : Saturate  UpperLimit=255  LowerLimit=-255
  Sum : Sum  Inputs=|+-
  Sum1 : Sum  Inputs=|+-
  VOLT----PWM : Gain  Gain=255/12
  wires:
  In1/1 -> Sum/1
  Gain1/1 -> 1/1
  Saturation2/1 -> Abs1/1
  PI2/1 -> VOLT----PWM/1  "u44"
  MATLAB Function/2(AIN2) -> AIN2/1  "ain2_4"
  Sum1/1 -> Gain1/1
  Gain/1 -> Sum1/1
  VOLT----PWM/1 -> MATLAB Function/1(pwmRaw), Saturation2/1  "pwm_raw4"
  Abs1/1 -> Round/1
  1/1 -> Sum/2  "current4"
  Sum/1 -> PI2/1  "e44"
  Round/1 -> PWM SİNYALİ/1  "pwm4"
  Constant1/1 -> Sum1/2
  MATLAB Function/1(AIN1) -> AIN1/1  "ain1_4"
  Data Type Conversion/1 -> Gain/1
  AKIM SENSÖRÜNDEN GELEN VERİ CH3/1 -> Data Type Conversion/1  "current_raw4"

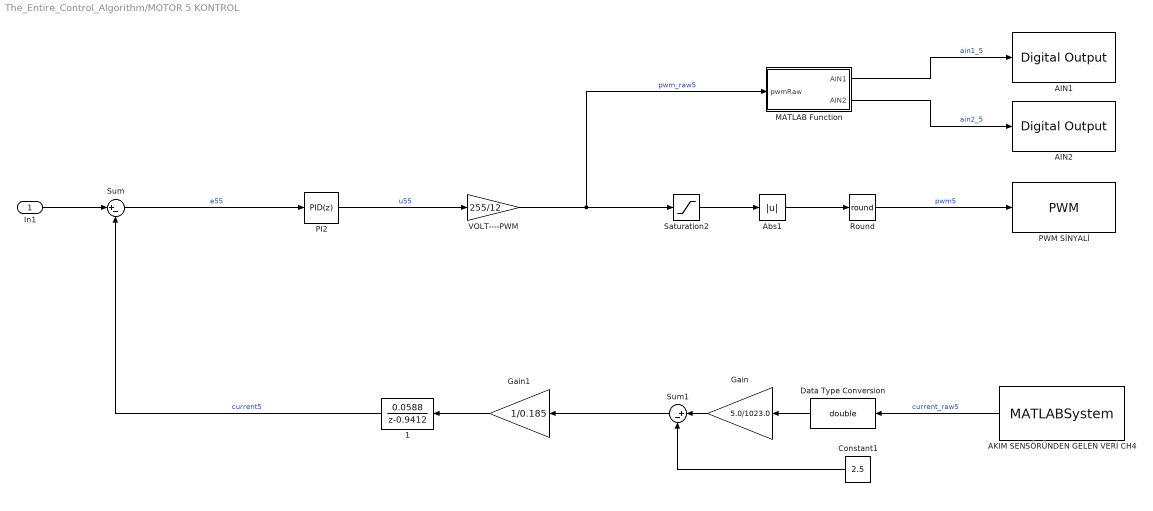
== system The_Entire_Control_Algorithm/MOTOR 5 KONTROL ==
  In1 : Inport
  1 : DiscreteTransferFcn  LoadFcn=dspblkCoreblockFVToolHelper(gcbh,'load');  Numerator=[0.0588]  Denominator=[1 -0.9412]
      settings: CopyFcn=dspblkCoreblockFVToolHelper(gcbh,'copy');  DeleteFcn=dspblkCoreblockFVToolHelper(gcbh,'close');  ModelCloseFcn=dspblkCoreblockFVToolHelper(gcbh,'close');  PreSaveFcn=dspblkCoreblockFVToolHelper(gcbh,'presave');  PostSaveFcn=dspblkCoreblockFVToolHelper(gcbh,'postsave');  CloseFcn=dspblkCoreblockFVToolHelper(gcbh,'close');
  AIN1 : arduinolib/Digital Output  pinNumber=32  Direction=output  blockPlatform=arduino
  AIN2 : arduinolib/Digital Output  pinNumber=33  Direction=output  blockPlatform=arduino
  AKIM SENSÖRÜNDEN GELEN VERİ CH4 : MATLABSystem  System=MCP3208Reader  Channel=0  SimulateUsing=Code generation
      mask Type: MCP3208Reader
      mask Display:
      | disp('MCP3208Reader');
      | port_label('output',1,'value');
  Abs1 : Abs  RndMeth=Round  SaturateOnIntegerOverflow=off
  Constant1 : Constant  Value=2.5
  Data Type Conversion : DataTypeConversion  OutDataTypeStr=double  SaturateOnIntegerOverflow=off  RndMeth=Floor
  Gain : Gain  Gain=5.0/1023.0
  Gain1 : Gain  Gain=1/0.185
  MATLAB Function : MATLAB Function  TreatAsAtomicUnit=on
  PI2 : slpidlib/PID Controller  Controller=PID  Form=Parallel  TimeDomain=Discrete-time  UseExternalTs=off  SampleTime=0.001  IntegratorMethod=Forward Euler  FilterMethod=Forward Euler  ControllerParametersSource=internal  P=21  I=900  UseKiTs=off  D=0.15  UseExternalDerivativeSource=off  N=100  UseFilter=off  TunerSelectOption=Transfer Function Based (PID Tuner App)  InitialConditionSource=internal  InitialConditionForIntegrator=0  InitialConditionForFilter=0  DifferentiatorICPrevScaledInput=0  ExternalReset=none  TrackingMode=off  Kt=1  LimitOutput=off  SatLimitsSource=internal  UpperSaturationLimit=inf  LowerSaturationLimit=-inf  LinearizeAsGain=on  AntiWindupMode=none  Kb=1  LimitIntegrator=off  UpperIntegratorSaturationLimit=inf  LowerIntegratorSaturationLimit=-inf  POutMin=[]  POutMax=[]  IOutMin=[]  IOutMax=[]  DOutMin=[]  DOutMax=[]  NOutMin=[]  NOutMax=[]  SumOutMin=[]  SumOutMax=[]  SaturationOutMin=[]  SaturationOutMax=[]  PParamMin=[]  PParamMax=[]  IParamMin=[]  IParamMax=[]  DParamMin=[]  DParamMax=[]  NParamMin=[]  NParamMax=[]  KbParamMin=[]  KbParamMax=[]  KtParamMin=[]  KtParamMax=[]  KbOutMin=[]  KbOutMax=[]  KtOutMin=[]  KtOutMax=[]  IntegratorOutMin=[]  IntegratorOutMax=[]  FilterOutMin=[]  FilterOutMax=[]  SumI1OutMin=[]  SumI1OutMax=[]  SumI2OutMin=[]  SumI2OutMax=[]  SumI3OutMin=[]  SumI3OutMax=[]  SumI4OutMin=[]  SumI4OutMax=[]  SumDOutMin=[]  SumDOutMax=[]  DifferentiatorOutMin=[]  DifferentiatorOutMax=[]  FilterDiffOutCoefMin=[]  FilterDiffOutCoefMax=[]  ReciprocalOutMin=[]  ReciprocalOutMax=[]  SumDenOutMin=[]  SumDenOutMax=[]  SumNumOutMin=[]  SumNumOutMax=[]  DivideOutMin=[]  DivideOutMax=[]  UdiffTsProdOutMin=[]  UdiffTsProdOutMax=[]  NTsProdOutMin=[]  NTsProdOutMax=[]  UintegralTsProdOutMin=[]  UintegralTsProdOutMax=[]  UngainTsProdOutMin=[]  UngainTsProdOutMax=[]  ClampingZeroOutDataTypeStr=Inherit: Inherit via back propagation  ClampingZeroOutMin=[]  ClampingZeroOutMax=[]  FilterDenConstantOutDataTypeStr=Inherit: Inherit via back propagation  FilterDenConstantOutMin=[]  FilterDenConstantOutMax=[]  PCopyOutDataTypeStr=Inherit: Inherit via back propagation  PCopyOutMin=[]  PCopyOutMax=[]  NCopyOutDataTypeStr=Inherit: Inherit via back propagation  NCopyOutMin=[]  NCopyOutMax=[]  IntegratorContinuousStateAttributes=''  IntegratorStateMustResolveToSignalObject=off  IntegratorRTWStateStorageClass=Auto  FilterContinuousStateAttributes=''  FilterStateMustResolveToSignalObject=off  FilterRTWStateStorageClass=Auto  ParallelPVariant=InternalParameters  IdealPVariant=Disabled  IVariant=InternalParameters  DVariant=InternalParameters  IntegratorVariant=Discrete  SatVariant=Disabled  AWVariant=Passthrough  PCopyVariant=Disabled  TRVariant=Disabled  FdbkBlocksVariant=Forward  IdealPFdbkVariant=Disabled  SatFdbkVariant=Disabled  DerivativeFilterVariant=Differentiator  NVariant=Passthrough  NCopyVariant=Disabled_SignalSpec  FilterICVariant=InternalICsDifferentiator  IntegratorICVariant=InternalICs  ExternalResetVariant=Disabled  TRSumVariant=Passthrough  SumFdbkVariant=Disabled  SumVariant=Sum_PID  TsampFilterVariant=InternalTs  TsampNgainVariant=Passthrough  TsampIntegralVariant=Disabled_SignalSpec  ExternalSaturationOutDataTypeStr=Inherit: Same as second input  DerivativeSourceVariant=ErrorSignal  PreIntVariant=InternalPreInt
  PWM SİNYALİ : arduinolib/PWM  pinNumber=6  frequencyType=Default  desiredFrequency=490  achievableFrequency=490.2
  Round : Rounding  Operator=round
  Saturation2 : Saturate  UpperLimit=255  LowerLimit=-255
  Sum : Sum  Inputs=|+-
  Sum1 : Sum  Inputs=|+-
  VOLT----PWM : Gain  Gain=255/12
  wires:
  In1/1 -> Sum/1
  MATLAB Function/2(AIN2) -> AIN2/1  "ain2_5"
  Gain1/1 -> 1/1
  PI2/1 -> VOLT----PWM/1  "u55"
  Saturation2/1 -> Abs1/1
  Constant1/1 -> Sum1/2
  MATLAB Function/1(AIN1) -> AIN1/1  "ain1_5"
  Round/1 -> PWM SİNYALİ/1  "pwm5"
  1/1 -> Sum/2  "current5"
  Gain/1 -> Sum1/1
  Sum/1 -> PI2/1  "e55"
  VOLT----PWM/1 -> MATLAB Function/1(pwmRaw), Saturation2/1  "pwm_raw5"
  Sum1/1 -> Gain1/1
  Abs1/1 -> Round/1
  Data Type Conversion/1 -> Gain/1
  AKIM SENSÖRÜNDEN GELEN VERİ CH4/1 -> Data Type Conversion/1  "current_raw5"

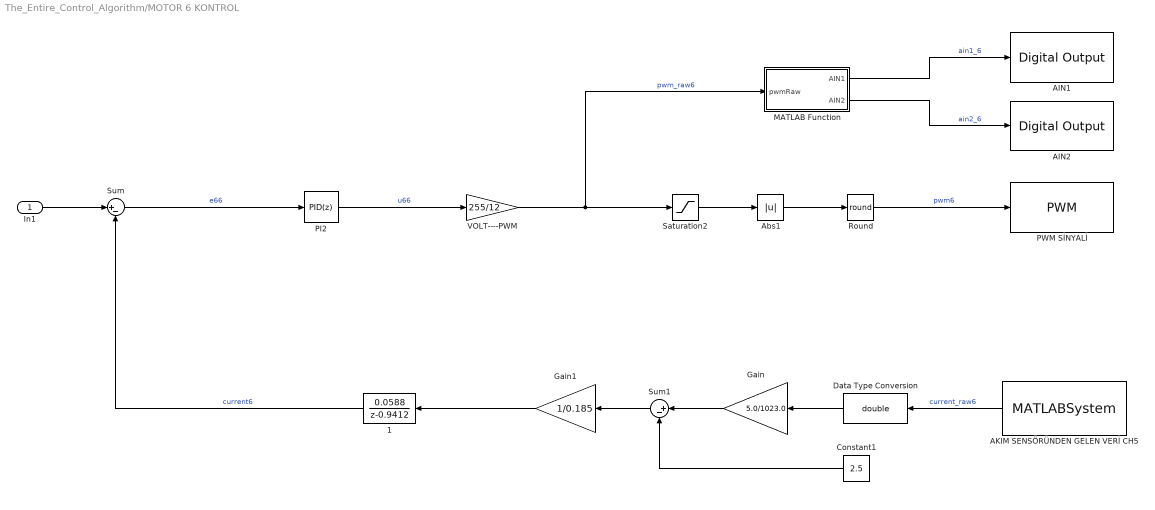
== system The_Entire_Control_Algorithm/MOTOR 6 KONTROL ==
  In1 : Inport
  1 : DiscreteTransferFcn  LoadFcn=dspblkCoreblockFVToolHelper(gcbh,'load');  Numerator=[0.0588]  Denominator=[1 -0.9412]
      settings: CopyFcn=dspblkCoreblockFVToolHelper(gcbh,'copy');  DeleteFcn=dspblkCoreblockFVToolHelper(gcbh,'close');  ModelCloseFcn=dspblkCoreblockFVToolHelper(gcbh,'close');  PreSaveFcn=dspblkCoreblockFVToolHelper(gcbh,'presave');  PostSaveFcn=dspblkCoreblockFVToolHelper(gcbh,'postsave');  CloseFcn=dspblkCoreblockFVToolHelper(gcbh,'close');
  AIN1 : arduinolib/Digital Output  pinNumber=34  Direction=output  blockPlatform=arduino
  AIN2 : arduinolib/Digital Output  pinNumber=35  Direction=output  blockPlatform=arduino
  AKIM SENSÖRÜNDEN GELEN VERİ CH5 : MATLABSystem  System=MCP3208Reader  Channel=0  SimulateUsing=Code generation
      mask Type: MCP3208Reader
      mask Display:
      | disp('MCP3208Reader');
      | port_label('output',1,'value');
  Abs1 : Abs  RndMeth=Round  SaturateOnIntegerOverflow=off
  Constant1 : Constant  Value=2.5
  Data Type Conversion : DataTypeConversion  OutDataTypeStr=double  SaturateOnIntegerOverflow=off  RndMeth=Floor
  Gain : Gain  Gain=5.0/1023.0
  Gain1 : Gain  Gain=1/0.185
  MATLAB Function : MATLAB Function  TreatAsAtomicUnit=on
  PI2 : slpidlib/PID Controller  Controller=PID  Form=Parallel  TimeDomain=Discrete-time  UseExternalTs=off  SampleTime=0.001  IntegratorMethod=Forward Euler  FilterMethod=Forward Euler  ControllerParametersSource=internal  P=21  I=900  UseKiTs=off  D=0.15  UseExternalDerivativeSource=off  N=100  UseFilter=off  TunerSelectOption=Transfer Function Based (PID Tuner App)  InitialConditionSource=internal  InitialConditionForIntegrator=0  InitialConditionForFilter=0  DifferentiatorICPrevScaledInput=0  ExternalReset=none  TrackingMode=off  Kt=1  LimitOutput=off  SatLimitsSource=internal  UpperSaturationLimit=inf  LowerSaturationLimit=-inf  LinearizeAsGain=on  AntiWindupMode=none  Kb=1  LimitIntegrator=off  UpperIntegratorSaturationLimit=inf  LowerIntegratorSaturationLimit=-inf  POutMin=[]  POutMax=[]  IOutMin=[]  IOutMax=[]  DOutMin=[]  DOutMax=[]  NOutMin=[]  NOutMax=[]  SumOutMin=[]  SumOutMax=[]  SaturationOutMin=[]  SaturationOutMax=[]  PParamMin=[]  PParamMax=[]  IParamMin=[]  IParamMax=[]  DParamMin=[]  DParamMax=[]  NParamMin=[]  NParamMax=[]  KbParamMin=[]  KbParamMax=[]  KtParamMin=[]  KtParamMax=[]  KbOutMin=[]  KbOutMax=[]  KtOutMin=[]  KtOutMax=[]  IntegratorOutMin=[]  IntegratorOutMax=[]  FilterOutMin=[]  FilterOutMax=[]  SumI1OutMin=[]  SumI1OutMax=[]  SumI2OutMin=[]  SumI2OutMax=[]  SumI3OutMin=[]  SumI3OutMax=[]  SumI4OutMin=[]  SumI4OutMax=[]  SumDOutMin=[]  SumDOutMax=[]  DifferentiatorOutMin=[]  DifferentiatorOutMax=[]  FilterDiffOutCoefMin=[]  FilterDiffOutCoefMax=[]  ReciprocalOutMin=[]  ReciprocalOutMax=[]  SumDenOutMin=[]  SumDenOutMax=[]  SumNumOutMin=[]  SumNumOutMax=[]  DivideOutMin=[]  DivideOutMax=[]  UdiffTsProdOutMin=[]  UdiffTsProdOutMax=[]  NTsProdOutMin=[]  NTsProdOutMax=[]  UintegralTsProdOutMin=[]  UintegralTsProdOutMax=[]  UngainTsProdOutMin=[]  UngainTsProdOutMax=[]  ClampingZeroOutDataTypeStr=Inherit: Inherit via back propagation  ClampingZeroOutMin=[]  ClampingZeroOutMax=[]  FilterDenConstantOutDataTypeStr=Inherit: Inherit via back propagation  FilterDenConstantOutMin=[]  FilterDenConstantOutMax=[]  PCopyOutDataTypeStr=Inherit: Inherit via back propagation  PCopyOutMin=[]  PCopyOutMax=[]  NCopyOutDataTypeStr=Inherit: Inherit via back propagation  NCopyOutMin=[]  NCopyOutMax=[]  IntegratorContinuousStateAttributes=''  IntegratorStateMustResolveToSignalObject=off  IntegratorRTWStateStorageClass=Auto  FilterContinuousStateAttributes=''  FilterStateMustResolveToSignalObject=off  FilterRTWStateStorageClass=Auto  ParallelPVariant=InternalParameters  IdealPVariant=Disabled  IVariant=InternalParameters  DVariant=InternalParameters  IntegratorVariant=Discrete  SatVariant=Disabled  AWVariant=Passthrough  PCopyVariant=Disabled  TRVariant=Disabled  FdbkBlocksVariant=Forward  IdealPFdbkVariant=Disabled  SatFdbkVariant=Disabled  DerivativeFilterVariant=Differentiator  NVariant=Passthrough  NCopyVariant=Disabled_SignalSpec  FilterICVariant=InternalICsDifferentiator  IntegratorICVariant=InternalICs  ExternalResetVariant=Disabled  TRSumVariant=Passthrough  SumFdbkVariant=Disabled  SumVariant=Sum_PID  TsampFilterVariant=InternalTs  TsampNgainVariant=Passthrough  TsampIntegralVariant=Disabled_SignalSpec  ExternalSaturationOutDataTypeStr=Inherit: Same as second input  DerivativeSourceVariant=ErrorSignal  PreIntVariant=InternalPreInt
  PWM SİNYALİ : arduinolib/PWM  pinNumber=7  frequencyType=Default  desiredFrequency=490  achievableFrequency=490.2
  Round : Rounding  Operator=round
  Saturation2 : Saturate  UpperLimit=255  LowerLimit=-255
  Sum : Sum  Inputs=|+-
  Sum1 : Sum  Inputs=|+-
  VOLT----PWM : Gain  Gain=255/12
  wires:
  In1/1 -> Sum/1
  Sum1/1 -> Gain1/1
  Abs1/1 -> Round/1
  VOLT----PWM/1 -> MATLAB Function/1(pwmRaw), Saturation2/1  "pwm_raw6"
  Sum/1 -> PI2/1  "e66"
  Gain/1 -> Sum1/1
  1/1 -> Sum/2  "current6"
  Gain1/1 -> 1/1
  Constant1/1 -> Sum1/2
  PI2/1 -> VOLT----PWM/1  "u66"
  Saturation2/1 -> Abs1/1
  MATLAB Function/1(AIN1) -> AIN1/1  "ain1_6"
  MATLAB Function/2(AIN2) -> AIN2/1  "ain2_6"
  Round/1 -> PWM SİNYALİ/1  "pwm6"
  Data Type Conversion/1 -> Gain/1
  AKIM SENSÖRÜNDEN GELEN VERİ CH5/1 -> Data Type Conversion/1  "current_raw6"

== system The_Entire_Control_Algorithm/EMPEDANS KONTROL2/Discrete_Derivative1 ==
  In1 : Inport
  {1..3,5} (4 alike) : DiscreteTransferFcn  LoadFcn=dspblkCoreblockFVToolHelper(gcbh,'load');  Numerator=[0.0588]  Denominator=[1 -0.9412]
      settings: CopyFcn=dspblkCoreblockFVToolHelper(gcbh,'copy');  DeleteFcn=dspblkCoreblockFVToolHelper(gcbh,'close');  ModelCloseFcn=dspblkCoreblockFVToolHelper(gcbh,'close');  PreSaveFcn=dspblkCoreblockFVToolHelper(gcbh,'presave');  PostSaveFcn=dspblkCoreblockFVToolHelper(gcbh,'postsave');  CloseFcn=dspblkCoreblockFVToolHelper(gcbh,'close');
  Discrete Derivative : simulink/Discrete/Discrete Derivative  gainval=1.0  ICPrevScaledInput=0.0  InputProcessing=Columns as channels (frame based)  OutMin=[]  OutMax=[]  OutDataType=fixdt(1, 16)  OutScaling=2^-10  DoSatur=off
  Out1 : Outport
  wires:
  Discrete Derivative/1 -> 5/1
  5/1 -> 1/1
  3/1 -> 2/1
  1/1 -> 3/1
  2/1 -> Out1/1
  In1/1 -> Discrete Derivative/1

== system The_Entire_Control_Algorithm/EMPEDANS KONTROL2/Discrete_Derivative2 ==
  In1 : Inport
  {1..3,5} (4 alike) : DiscreteTransferFcn  LoadFcn=dspblkCoreblockFVToolHelper(gcbh,'load');  Numerator=[0.0588]  Denominator=[1 -0.9412]
      settings: CopyFcn=dspblkCoreblockFVToolHelper(gcbh,'copy');  DeleteFcn=dspblkCoreblockFVToolHelper(gcbh,'close');  ModelCloseFcn=dspblkCoreblockFVToolHelper(gcbh,'close');  PreSaveFcn=dspblkCoreblockFVToolHelper(gcbh,'presave');  PostSaveFcn=dspblkCoreblockFVToolHelper(gcbh,'postsave');  CloseFcn=dspblkCoreblockFVToolHelper(gcbh,'close');
  Discrete Derivative : simulink/Discrete/Discrete Derivative  gainval=1.0  ICPrevScaledInput=0.0  InputProcessing=Columns as channels (frame based)  OutMin=[]  OutMax=[]  OutDataType=fixdt(1, 16)  OutScaling=2^-10  DoSatur=off
  Out1 : Outport
  wires:
  In1/1 -> Discrete Derivative/1
  Discrete Derivative/1 -> 5/1
  5/1 -> 1/1
  3/1 -> 2/1
  1/1 -> 3/1
  2/1 -> Out1/1

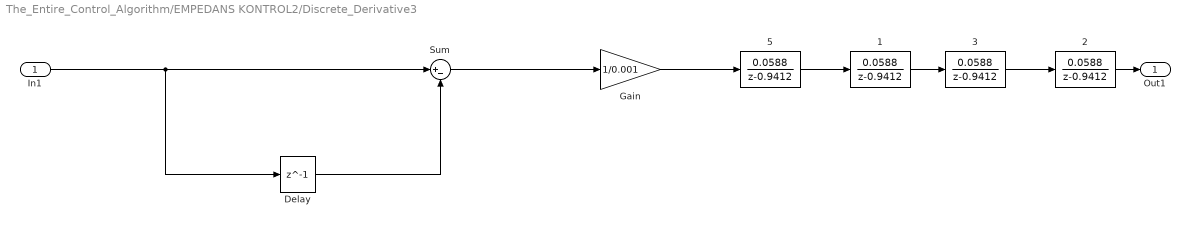
== system The_Entire_Control_Algorithm/EMPEDANS KONTROL2/Discrete_Derivative3 ==
  In1 : Inport
  {1..3,5} (4 alike) : DiscreteTransferFcn  LoadFcn=dspblkCoreblockFVToolHelper(gcbh,'load');  Numerator=[0.0588]  Denominator=[1 -0.9412]
      settings: CopyFcn=dspblkCoreblockFVToolHelper(gcbh,'copy');  DeleteFcn=dspblkCoreblockFVToolHelper(gcbh,'close');  ModelCloseFcn=dspblkCoreblockFVToolHelper(gcbh,'close');  PreSaveFcn=dspblkCoreblockFVToolHelper(gcbh,'presave');  PostSaveFcn=dspblkCoreblockFVToolHelper(gcbh,'postsave');  CloseFcn=dspblkCoreblockFVToolHelper(gcbh,'close');
  Delay : Delay  DelayLength=1  InputProcessing=Columns as channels (frame based)  SampleTime=0.001
  Gain : Gain  Gain=1/0.001
  Sum : Sum  Inputs=|+-
  Out1 : Outport
  wires:
  In1/1 -> Sum/1, Delay/1
  Delay/1 -> Sum/2
  Sum/1 -> Gain/1
  Gain/1 -> 5/1
  5/1 -> 1/1
  3/1 -> 2/1
  1/1 -> 3/1
  2/1 -> Out1/1

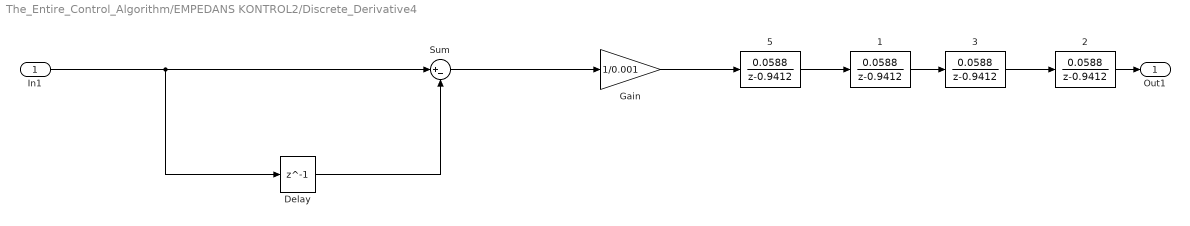
== system The_Entire_Control_Algorithm/EMPEDANS KONTROL2/Discrete_Derivative4 ==
  In1 : Inport
  {1..3,5} (4 alike) : DiscreteTransferFcn  LoadFcn=dspblkCoreblockFVToolHelper(gcbh,'load');  Numerator=[0.0588]  Denominator=[1 -0.9412]
      settings: CopyFcn=dspblkCoreblockFVToolHelper(gcbh,'copy');  DeleteFcn=dspblkCoreblockFVToolHelper(gcbh,'close');  ModelCloseFcn=dspblkCoreblockFVToolHelper(gcbh,'close');  PreSaveFcn=dspblkCoreblockFVToolHelper(gcbh,'presave');  PostSaveFcn=dspblkCoreblockFVToolHelper(gcbh,'postsave');  CloseFcn=dspblkCoreblockFVToolHelper(gcbh,'close');
  Delay : Delay  DelayLength=1  InputProcessing=Columns as channels (frame based)  SampleTime=0.001
  Gain : Gain  Gain=1/0.001
  Sum : Sum  Inputs=|+-
  Out1 : Outport
  wires:
  In1/1 -> Sum/1, Delay/1
  Delay/1 -> Sum/2
  Sum/1 -> Gain/1
  Gain/1 -> 5/1
  5/1 -> 1/1
  3/1 -> 2/1
  1/1 -> 3/1
  2/1 -> Out1/1

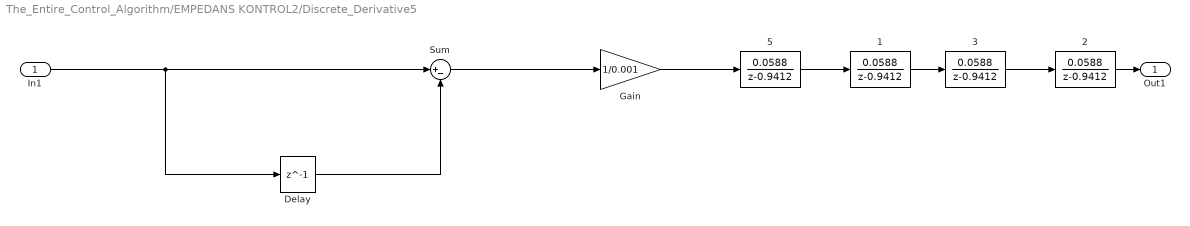
== system The_Entire_Control_Algorithm/EMPEDANS KONTROL2/Discrete_Derivative5 ==
  In1 : Inport
  {1..3,5} (4 alike) : DiscreteTransferFcn  LoadFcn=dspblkCoreblockFVToolHelper(gcbh,'load');  Numerator=[0.0588]  Denominator=[1 -0.9412]
      settings: CopyFcn=dspblkCoreblockFVToolHelper(gcbh,'copy');  DeleteFcn=dspblkCoreblockFVToolHelper(gcbh,'close');  ModelCloseFcn=dspblkCoreblockFVToolHelper(gcbh,'close');  PreSaveFcn=dspblkCoreblockFVToolHelper(gcbh,'presave');  PostSaveFcn=dspblkCoreblockFVToolHelper(gcbh,'postsave');  CloseFcn=dspblkCoreblockFVToolHelper(gcbh,'close');
  Delay : Delay  DelayLength=1  InputProcessing=Columns as channels (frame based)  SampleTime=0.001
  Gain : Gain  Gain=1/0.001
  Sum : Sum  Inputs=|+-
  Out1 : Outport
  wires:
  In1/1 -> Sum/1, Delay/1
  Delay/1 -> Sum/2
  Sum/1 -> Gain/1
  Gain/1 -> 5/1
  5/1 -> 1/1
  3/1 -> 2/1
  1/1 -> 3/1
  2/1 -> Out1/1

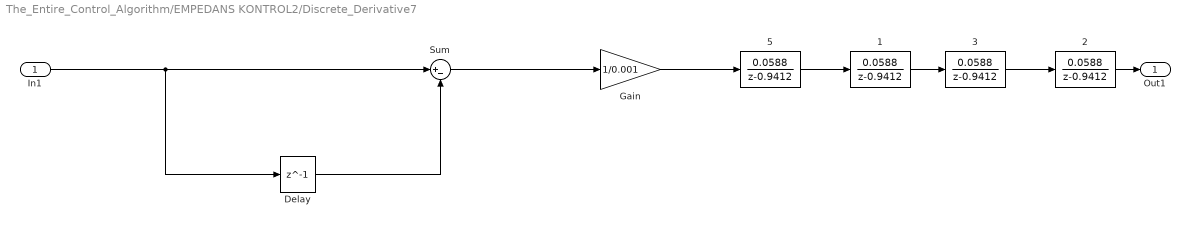
== system The_Entire_Control_Algorithm/EMPEDANS KONTROL2/Discrete_Derivative7 ==
  In1 : Inport
  {1..3,5} (4 alike) : DiscreteTransferFcn  LoadFcn=dspblkCoreblockFVToolHelper(gcbh,'load');  Numerator=[0.0588]  Denominator=[1 -0.9412]
      settings: CopyFcn=dspblkCoreblockFVToolHelper(gcbh,'copy');  DeleteFcn=dspblkCoreblockFVToolHelper(gcbh,'close');  ModelCloseFcn=dspblkCoreblockFVToolHelper(gcbh,'close');  PreSaveFcn=dspblkCoreblockFVToolHelper(gcbh,'presave');  PostSaveFcn=dspblkCoreblockFVToolHelper(gcbh,'postsave');  CloseFcn=dspblkCoreblockFVToolHelper(gcbh,'close');
  Delay : Delay  DelayLength=1  InputProcessing=Columns as channels (frame based)  SampleTime=0.001
  Gain : Gain  Gain=1/0.001
  Sum : Sum  Inputs=|+-
  Out1 : Outport
  wires:
  In1/1 -> Sum/1, Delay/1
  Delay/1 -> Sum/2
  Sum/1 -> Gain/1
  Gain/1 -> 5/1
  5/1 -> 1/1
  3/1 -> 2/1
  1/1 -> 3/1
  2/1 -> Out1/1
